simulink model "KaplunenkoDD_Task1v1corr"  (R2020a)
settings: Solver=VariableStepAuto  StartTime=0.0  StopTime=45  RelTol=1e-3  EnableMultiTasking=on
libraries: simulink x2
settings Model: Creator=Boris  LastModifiedBy=Dmitry Kaplunenko
settings DataIOCC: SaveOutput=off  SignalLogging=off  DSMLogging=off  SaveTime=off  ReturnWorkspaceOutputs=off
settings OptimizationCC: LifeSpan=inf
settings DebuggingCC: SFUnexpectedBacktrackingDiag=warning  SFNoUnconditionalDefaultTransitionDiag=warning  SFExecutionAtInitializationDiag=none  ArithmeticOperatorsInVariantConditions=warning
settings SFSimCC: SimUseLocalCustomCode=off  CustomCodeUndefinedFunction=UseInterfaceOnly
settings RTWCC: RTWUseLocalCustomCode=off
settings CodeAppCC: StateflowObjectComments=on
settings GRTTargetCC: TargetLangStandard=C89/C90 (ANSI)
settings ConfigComp: CovMetricSettings=dw  CovHtmlReporting=on  CovSaveCumulativeToWorkspaceVar=on  CovSaveSingleToWorkspaceVar=on  CovExternalEMLEnable=off

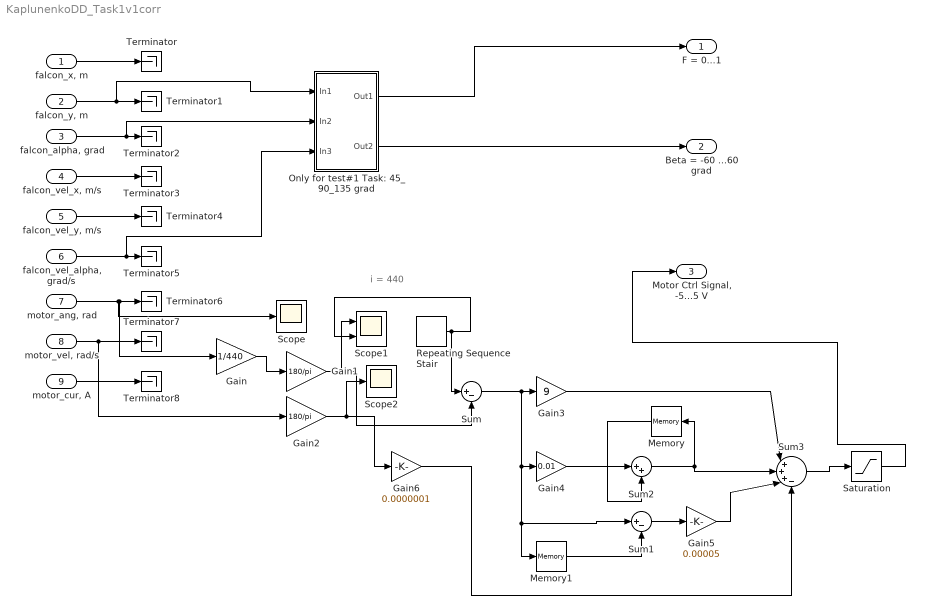
== system KaplunenkoDD_Task1v1corr ==
  note: i = 440
  "falcon_x, m" : Inport  OutDataTypeStr=double  PortDimensions=1  SampleTime=[0.01,0]
  "falcon_y, m" : Inport  Port=2  OutDataTypeStr=double  PortDimensions=1  SampleTime=[0.01,0]
  "falcon_alpha, grad" : Inport  Port=3  OutDataTypeStr=double  PortDimensions=1  SampleTime=[0.01,0]
  "falcon_vel_x, m/s" : Inport  Port=4  OutDataTypeStr=double  PortDimensions=1  SampleTime=[0.01,0]
  "falcon_vel_y, m/s" : Inport  Port=5  OutDataTypeStr=double  PortDimensions=1  SampleTime=[0.01,0]
  "falcon_vel_alpha, grad/s" : Inport  Port=6  OutDataTypeStr=double  PortDimensions=1  SampleTime=[0.01,0]
  "motor_ang, rad" : Inport  Port=7  OutDataTypeStr=double  PortDimensions=1  SampleTime=[0.01,0]
  "motor_vel, rad/s" : Inport  Port=8  OutDataTypeStr=double  PortDimensions=1  SampleTime=[0.01,0]
  "motor_cur, A" : Inport  Port=9  OutDataTypeStr=double  PortDimensions=1  SampleTime=[0.01,0]
  Gain : Gain  Gain=1/440
  Gain1 : Gain  Gain=180/pi
  Gain2 : Gain  Gain=180/pi
  Gain3 : Gain  Gain=9
  Gain4 : Gain  Gain=0.01
  Gain5 : Gain  Gain=0.00005
  Gain6 : Gain  Gain=0.0000001
  Memory : Memory
  Memory1 : Memory
  Only for test#1 Task: 45_90_135 grad : Subsystem
  Repeating Sequence Stair : simulink/Sources/Repeating Sequence Stair  OutValues=[45 90 135].'  tsamp=15  OutMin=[]  OutMax=[]  OutDataTypeStr=double  OutputDataTypeScalingMode=double  OutDataType=fixdt(0,8)  ConRadixGroup=Best Precision: Vector-wise  OutScaling=2^-12
  Saturation : Saturate  UpperLimit=5  LowerLimit=-5
  Scope : Scope
  Scope1 : Scope  NumInputPorts=2
  Scope2 : Scope
  Sum : Sum  Inputs=|+-
  Sum1 : Sum  Inputs=|+-
  Sum2 : Sum  Inputs=|++
  Sum3 : Sum  Inputs=|+++-
  Terminator{,1..8} (9 alike) : Terminator
  F = 0...1 : Outport  OutDataTypeStr=double  PortDimensions=1  SampleTime=[0.01,0]  VectorParamsAs1DForOutWhenUnconnected=off
  Beta = -60 ...60 grad : Outport  Port=2  OutDataTypeStr=double  PortDimensions=1  SampleTime=[0.01,0]  VectorParamsAs1DForOutWhenUnconnected=off
  "Motor Ctrl Signal, -5...5 V" : Outport  Port=3  OutDataTypeStr=double  PortDimensions=1  SampleTime=[0,1]  VectorParamsAs1DForOutWhenUnconnected=off
  wires:
  "motor_ang, rad"/1 -> Scope/1, Terminator6/1, Gain/1
  "falcon_vel_y, m/s"/1 -> Terminator4/1
  "falcon_vel_x, m/s"/1 -> Terminator3/1
  "falcon_alpha, grad"/1 -> Terminator2/1, Only for test#1 Task: 45_90_135 grad/2(In2)
  "falcon_y, m"/1 -> Terminator1/1, Only for test#1 Task: 45_90_135 grad/1(In1)
  "falcon_x, m"/1 -> Terminator/1
  "motor_vel, rad/s"/1 -> Terminator7/1, Gain2/1
  "motor_cur, A"/1 -> Terminator8/1
  "falcon_vel_alpha, grad/s"/1 -> Terminator5/1, Only for test#1 Task: 45_90_135 grad/3(In3)
  Only for test#1 Task: 45_90_135 grad/1(Out1) -> F = 0...1/1
  Only for test#1 Task: 45_90_135 grad/2(Out2) -> Beta = -60 ...60 grad/1
  Gain/1 -> Gain1/1
  Gain1/1 -> Scope1/1, Sum/2
  Gain2/1 -> Scope2/1, Gain6/1
  Repeating Sequence Stair/1 -> Scope1/2, Sum/1
  Sum/1 -> Gain3/1, Gain4/1, Memory1/1, Sum1/1
  Gain4/1 -> Sum2/1
  Gain3/1 -> Sum3/1
  Sum2/1 -> Sum3/2, Memory/1
  Memory/1 -> Sum2/2
  Memory1/1 -> Sum1/2
  Sum1/1 -> Gain5/1
  Gain5/1 -> Sum3/3
  Sum3/1 -> Saturation/1
  Saturation/1 -> "Motor Ctrl Signal, -5...5 V"/1
  Gain6/1 -> Sum3/4

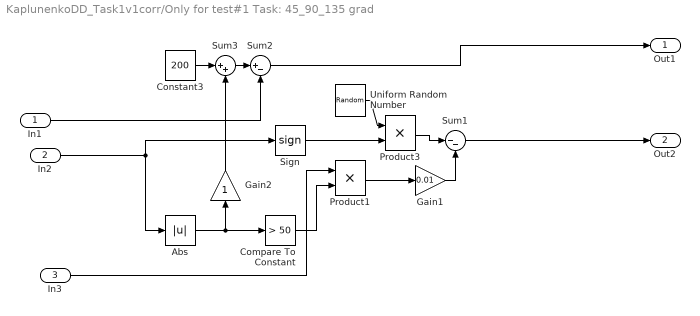
== system KaplunenkoDD_Task1v1corr/Only for test#1 Task: 45_90_135 grad ==
  In1 : Inport
  In2 : Inport  Port=2
  In3 : Inport  Port=3
  Abs : Abs
  Compare To Constant : simulink/Logic and Bit Operations/Compare To Constant  relop=>  const=50  OutDataTypeStr=boolean
  Constant3 : Constant  Value=200
  Gain1 : Gain  Gain=0.01
  Gain2 : Gain
  Product1 : Product
  Product3 : Product
  Sign : Signum
  Sum1 : Sum  Inputs=|--
  Sum2 : Sum  Inputs=|+-
  Sum3 : Sum  Inputs=|++
  Uniform Random Number : UniformRandomNumber  Minimum=20  Maximum=60  SampleTime=5
  Out1 : Outport  VectorParamsAs1DForOutWhenUnconnected=off
  Out2 : Outport  Port=2  VectorParamsAs1DForOutWhenUnconnected=off
  wires:
  In3/1 -> Product1/1
  Sum1/1 -> Out2/1
  In1/1 -> Sum2/2
  Product3/1 -> Sum1/1
  In2/1 -> Abs/1, Sign/1
  Constant3/1 -> Sum3/1
  Gain2/1 -> Sum3/2
  Gain1/1 -> Sum1/2
  Sign/1 -> Product3/2
  Sum3/1 -> Sum2/1
  Uniform Random Number/1 -> Product3/1
  Sum2/1 -> Out1/1
  Abs/1 -> Gain2/1, Compare To Constant/1
  Product1/1 -> Gain1/1
  Compare To Constant/1 -> Product1/2
